simulink model "ThdRwRtStFwdBkwdIsPosChk"  (R2018b)
settings: Solver=FixedStepDiscrete  StartTime=0.0  StopTime=10.0  FixedStep=0.01  RelTol=1e-3
undefined symbols (not defined in the file or in its folder): KeSMSuThirdRwStFwdBkwdPosDelta_Val, KeSMSuThirdRwStFwdBkwdPosTolr_Val, KeSMSuVehicleModelConfig_Val
libraries: StIsPosChkLib x11, simulink x5
(part 2 of 2)

== system ThdRwRtStFwdBkwdIsPosChk/ThdRwRtStFwdBkwdIsPosChk_Cal_sys/Subsystem3/Subsystem8 ==
  PosV : Inport
  Pos : Inport  Port=2
  CalibArray : Inport  Port=3
  Delta : Inport  Port=4
  Tolr : Inport  Port=5
  XXStIsPos_Get : FunctionCaller  FunctionPrototype=[IsPos,IsPosZone,IsPosAlready] = XXStIsPos_Get(PosV,Pos,CalibArray,Delta,Tolr)  InputArgumentSpecifications=boolean(true), uint16(1), uint16([1;1;1]), uint16(1), uint16(1)  OutputArgumentSpecifications=boolean(true), boolean(true), boolean(true)
  IsPos : Outport
  IsPosZone : Outport  Port=2
  IsPosAlready : Outport  Port=3
  wires:
  Pos/1 -> XXStIsPos_Get/2
  Delta/1 -> XXStIsPos_Get/4
  CalibArray/1 -> XXStIsPos_Get/3
  XXStIsPos_Get/2 -> IsPosZone/1
  XXStIsPos_Get/1 -> IsPos/1
  Tolr/1 -> XXStIsPos_Get/5
  XXStIsPos_Get/3 -> IsPosAlready/1
  PosV/1 -> XXStIsPos_Get/1

== system ThdRwRtStFwdBkwdIsPosChk/ThdRwRtStFwdBkwdIsPosChk_Cal_sys/Subsystem3/Subsystem9 ==
  PosV : Inport
  Pos : Inport  Port=2
  CalibArray : Inport  Port=3
  Delta : Inport  Port=4
  Tolr : Inport  Port=5
  XXStIsPos_Get : FunctionCaller  FunctionPrototype=[IsPos,IsPosZone,IsPosAlready] = XXStIsPos_Get(PosV,Pos,CalibArray,Delta,Tolr)  InputArgumentSpecifications=boolean(true), uint16(1), uint16([1;1;1]), uint16(1), uint16(1)  OutputArgumentSpecifications=boolean(true), boolean(true), boolean(true)
  IsPos : Outport
  IsPosZone : Outport  Port=2
  IsPosAlready : Outport  Port=3
  wires:
  PosV/1 -> XXStIsPos_Get/1
  XXStIsPos_Get/3 -> IsPosAlready/1
  Tolr/1 -> XXStIsPos_Get/5
  XXStIsPos_Get/1 -> IsPos/1
  XXStIsPos_Get/2 -> IsPosZone/1
  CalibArray/1 -> XXStIsPos_Get/3
  Delta/1 -> XXStIsPos_Get/4
  Pos/1 -> XXStIsPos_Get/2
